simulink model "ctrl5_2_3"  (R2013a)
settings: Solver=ode3  StartTime=0.0  StopTime=5  FixedStep=h  RelTol=1e-3
InitFcn:
  | global r;
  | global h;
  | global b0;
  | r=30;
  | h=1e-3;
  | b0=1;
settings Model: Creator=asus1  LastModifiedBy=asus1

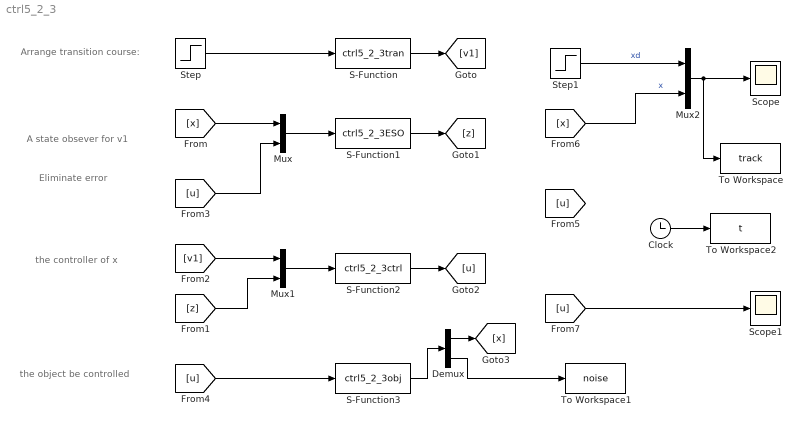
== system ctrl5_2_3 ==
  note: the object
      | be controlled
  note: the controller
      | of x
  note: Eliminate error
  note: A state obsever
      | for v1
  note: Arrange transition
      | course:
  Clock : Clock
  Demux : Demux  Outputs=2
  Mux : Mux  Inputs=2
  Mux1 : Mux  Inputs=2
  Mux2 : Mux  Inputs=2
  S-Function : S-Function  FunctionName=ctrl5_2_3tran  EnableBusSupport=off
  S-Function1 : S-Function  FunctionName=ctrl5_2_3ESO  EnableBusSupport=off
  S-Function2 : S-Function  FunctionName=ctrl5_2_3ctrl  EnableBusSupport=off
  S-Function3 : S-Function  FunctionName=ctrl5_2_3obj  EnableBusSupport=off
  Scope : Scope
      settings: YMin=0  YMax=1.1
  Scope1 : Scope
      settings: TimeRange=10  YMin=-2.25  YMax=2.25
  Step : Step  Time=0  SampleTime=0
  Step1 : Step  Time=0  SampleTime=0
  To Workspace : ToWorkspace  VariableName=track  SampleTime=-1
  To Workspace1 : ToWorkspace  VariableName=noise  SampleTime=-1
  To Workspace2 : ToWorkspace  VariableName=t  SampleTime=-1
  wires:
  Step/1 -> S-Function/1
  S-Function/1 -> [v1]
  S-Function1/1 -> [z]
  [u] -> Mux/2
  Mux/1 -> S-Function1/1
  [v1] -> Mux1/1
  [z] -> Mux1/2
  Mux1/1 -> S-Function2/1
  S-Function2/1 -> [u]
  [u] -> S-Function3/1
  [x] -> Mux/1
  Mux2/1 -> Scope/1, To Workspace/1
  [x] -> Mux2/2  "x"
  Step1/1 -> Mux2/1  "xd"
  [u] -> Scope1/1
  S-Function3/1 -> Demux/1
  Demux/1 -> [x]
  Demux/2 -> To Workspace1/1
  Clock/1 -> To Workspace2/1
